simulink subsystem "Motor"  (R2023a)
settings: Solver=VariableStepAuto  StartTime=0.0  StopTime=10.0  RelTol=1e-3
values from neighbouring files (symbols this model uses):
  J = 0.04    [main.m]
  km = 0.36    [main.m]
  kv = 0.45    [main.m]
  L = 0.01    [main.m]
  R = 0.5    [main.m]
settings Model: Creator=ycheb  LastModifiedBy=ycheb

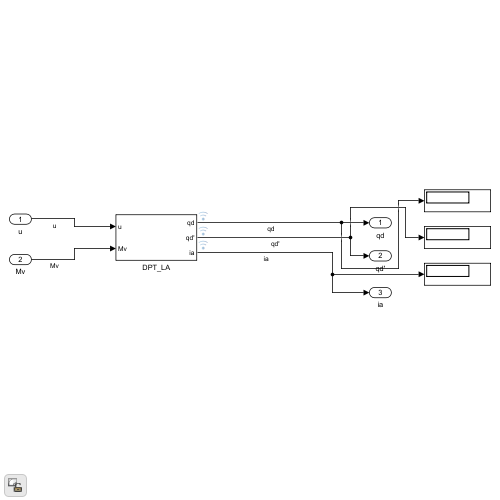
[thumbnail: Simulink's stored preview of the top-level diagram]
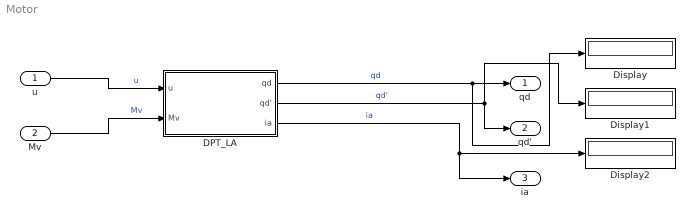
== system Motor ==
  u : Inport
  Mv : Inport  Port=2
  DPT_LA : Subsystem
  Display : Display
  Display1 : Display
  Display2 : Display
  qd : Outport
  qd' : Outport  Port=2
  ia : Outport  Port=3
  wires:
  DPT_LA/3(ia) -> Display2/1, ia/1  "ia"
  Mv/1 -> DPT_LA/2(Mv)  "Mv"
  DPT_LA/2(qd') -> Display1/1, qd'/1  "qd'"
  DPT_LA/1(qd) -> Display/1, qd/1  "qd"
  u/1 -> DPT_LA/1(u)  "u"

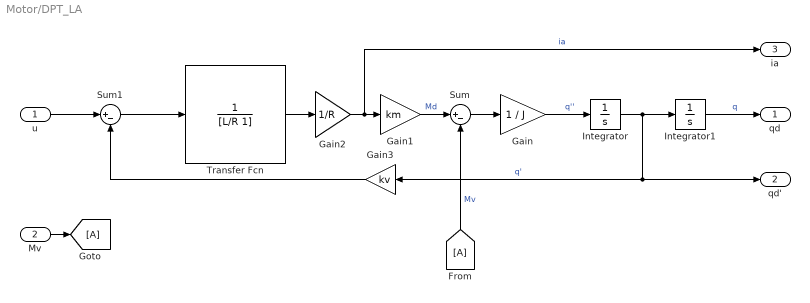
== system Motor/DPT_LA ==
  u : Inport
  Mv : Inport  Port=2
  From : From
  Gain : Gain  Gain=1 / J
  Gain1 : Gain  Gain=km
  Gain2 : Gain  Gain=1/R
  Gain3 : Gain  Gain=kv
  Goto : Goto
  Integrator : Integrator
  Integrator1 : Integrator
  Sum : Sum  Inputs=|+-
  Sum1 : Sum  Inputs=|+-
  Transfer Fcn : TransferFcn  Denominator=[L/R 1]
  qd : Outport
  qd' : Outport  Port=2
  ia : Outport  Port=3
  wires:
  Mv/1 -> Goto/1
  Sum1/1 -> Transfer Fcn/1
  Gain3/1 -> Sum1/2
  Transfer Fcn/1 -> Gain2/1
  Gain2/1 -> Gain1/1, ia/1  "ia"
  u/1 -> Sum1/1
  Gain1/1 -> Sum/1  "Md"
  From/1 -> Sum/2  "Mv"
  Sum/1 -> Gain/1
  Integrator1/1 -> qd/1  "q"
  Gain/1 -> Integrator/1  "q''"
  Integrator/1 -> Integrator1/1, Gain3/1, qd'/1  "q'"
